simulink model "gm_HSG"  (R2017b)
settings: Solver=FixedStepDiscrete  StartTime=0.0  StopTime=Ts_240p  RelTol=1e-3
InitFcn:
  | Ts = 1e-3;
  | Ts_240p = 402*324*Ts;
undefined symbols (not defined in the file): gray, Rec, SDTV
libraries: hdlsllib x15, visionhdlfilter x8, simulink x3, visionhdlio x2, visionhdlconversions x1, visionhdlanalysis x1, dspvision x1
settings Model: ModifiedByFormat=4mbilal@gmail.com  Creator=The MathWorks, Inc.  LastModifiedBy=4mbilal@gmail.com
settings DataIOCC: LimitDataPoints=on  SaveFormat=Array  SaveOutput=off  SaveTime=off
settings OptimizationCC: BlockReduction=off  ConditionallyExecuteInputs=off  DefaultParameterBehavior=Inlined  LifeSpan=inf
settings DebuggingCC: AlgebraicLoopMsg=error  SolverPrmCheckMsg=warning  InheritedTsInSrcMsg=none  SingleTaskRateTransMsg=error  ParameterPrecisionLossMsg=none  AllowSymbolicDim=off  SFUnexpectedBacktrackingDiag=warning  SFNoUnconditionalDefaultTransitionDiag=warning  SFExecutionAtInitializationDiag=none  IntegerSaturationMsg=none
settings HardwareCC: ProdBitPerPointer=32  ProdBitPerSizeT=32  ProdBitPerPtrDiffT=32  ProdLargestAtomicFloat=None  ProdIntDivRoundTo=Undefined  ProdEndianess=Unspecified  ProdWordSize=32  ProdHWDeviceType=ASIC/FPGA->ASIC/FPGA  ProdEqTarget=off
settings ModelReferenceCC: PropagateSignalLabelsOutOfModel=off
settings CodeAppCC: StateflowObjectComments=on
settings GRTTargetCC: TargetLangStandard=C89/C90 (ANSI)  GeneratePreprocessorConditionals=Disable all
settings ConfigComp: CovMetricSettings=dw  CovHtmlReporting=on  CovSaveCumulativeToWorkspaceVar=on  CovSaveSingleToWorkspaceVar=on  CovShowResultsExplorer=off  CovExternalEMLEnable=off  CovSFcnEnable=off

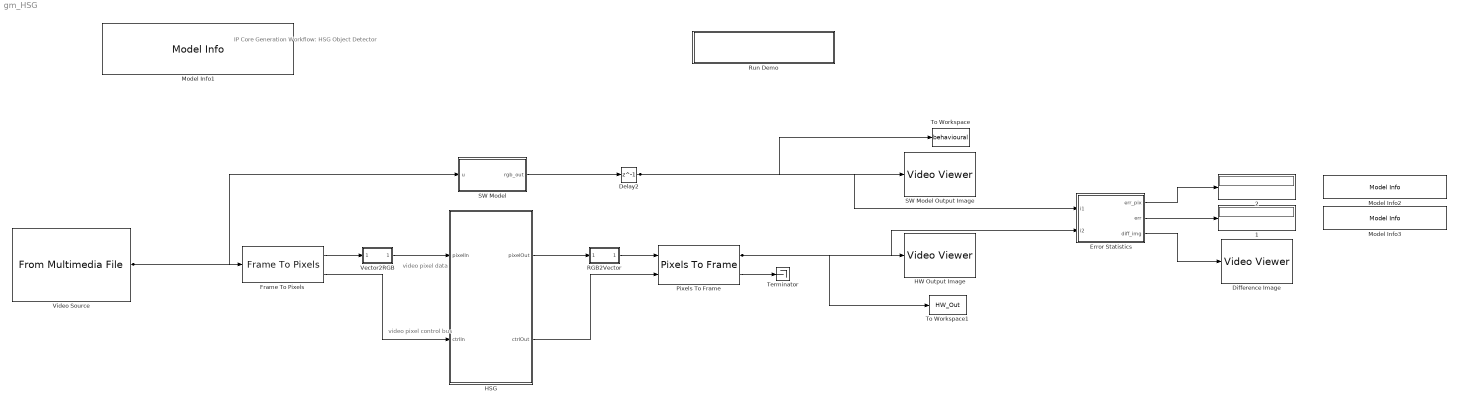
== system gm_HSG ==
  note: video pixel control bus
  note: IP Core Generation Workflow: HSG Object Detector
  note: video pixel data
  " 1" : Display
  " 2" : Display
  Delay2 : Delay  DelayLength=1  InitialCondition=0
  Difference Image : VideoViewer  colormapValue=gray(256)  FigPos=[516.2 717.2 730.4 340.8]
  Error Statistics : MATLAB Function  TreatAsAtomicUnit=on
  Frame To Pixels : visionhdlio/Frame To Pixels  NumComponents=3  VideoFormat=240p  ActivePixelsPerLine=32  ActiveVideoLines=18  TotalPixelsPerLine=42  TotalVideoLines=28  StartingActiveLine=6  FrontPorch=5  SampleTime=0
      settings: SourceProductName=Vision HDL Toolbox  SourceProductBaseCode=VT
  HSG : Subsystem  TreatAsAtomicUnit=on
  HW Output Image : VideoViewer  colormapValue=gray(256)  FigPos=[21.8 576.4 730.4 446.4]
  Model Info1 : simulink/Model-Wide Utilities/Model Info  Frame=on  DisplayStringWithTags=|  HorizontalTextAlignment=Center  LeftAlignmentValue=0.5
      | This Simulink model serves as the "High Level"
      |  framework for training, testing and HDL IP Core
      |  generation for video based object detection using
      |  HSG as the main feature.
  Model Info2 : simulink/Model-Wide Utilities/Model Info  Frame=on  DisplayStringWithTags=Percentage of Pixels with error  HorizontalTextAlignment=Center  LeftAlignmentValue=0.5
  Model Info3 : simulink/Model-Wide Utilities/Model Info  Frame=on  DisplayStringWithTags=Average error value per pixel  HorizontalTextAlignment=Center  LeftAlignmentValue=0.5
  Pixels To Frame : visionhdlio/Pixels To Frame  NumComponents=3  VideoFormat=240p  ActivePixelsPerLine=32  ActiveVideoLines=18  TotalPixelsPerLine=42  TotalVideoLines=28
      settings: SourceProductName=Vision HDL Toolbox  SourceProductBaseCode=VT
  RGB2Vector : Subsystem
  Run Demo : Subsystem
      settings: OpenFcn=hdladvisor([bdroot, '/HSG'])
      mask Display: disp('Launch HDL Workflow Advisor')
  SW Model : MATLAB Function  TreatAsAtomicUnit=on
  SW Model Output Image : VideoViewer  colormapValue=gray(256)  FigPos=[733.8 573.2 730.4 446.4]
  Terminator : Terminator
  To Workspace : ToWorkspace  VariableName=behavioural  SaveFormat=Timeseries  SampleTime=-1
  To Workspace1 : ToWorkspace  VariableName=HW_Out  SaveFormat=Timeseries  SampleTime=-1
  Vector2RGB : Subsystem
  Video Source : dspvision/From Multimedia File  inputFilename=E:\RnD\Current_Projects\Musawwir\Frameworks\HW\Musawwir_HW_Zedboard\Custom_IP_Cores\Matlab\HSG\engine_small.png  loop=on  numPlays=inf  outputStreams=Video only  videoDataType=uint8  audioDataType=int16  inheritSampleTime=off  userDefinedSampleTime=Ts_240p  noAudioOutput=off  isIntensityVideo=off  fourcc=RGB  colorVideoFormat=One multidimensional signal  outputEOF=off  dataOrg=Column-major  audioFrameSize=1024  computeAudioFrameSize=off  outSamplingMode=Sample based
      settings: SourceProductBaseCode=VP
  wires:
  Error Statistics/1(err_pix) -> " 2"/1
  Error Statistics/3(diff_img) -> Difference Image/1
  Delay2/1 -> SW Model Output Image/1, To Workspace/1, Error Statistics/1(i1)
  SW Model/1(rgb_out) -> Delay2/1
  Error Statistics/2(err) -> " 1"/1
  Pixels To Frame/1 -> HW Output Image/1, To Workspace1/1, Error Statistics/2(i2)
  Video Source/1 -> Frame To Pixels/1, SW Model/1(u)
  RGB2Vector/1(RGBVector) -> Pixels To Frame/1
  Frame To Pixels/2 -> HSG/2(ctrlIn)
  HSG/2(ctrlOut) -> Pixels To Frame/2
  Frame To Pixels/1 -> Vector2RGB/1(RGBVector)
  HSG/1(pixelOut) -> RGB2Vector/1(RGB)
  Vector2RGB/1(RGB) -> HSG/1(pixelIn)
  Pixels To Frame/2 -> Terminator/1

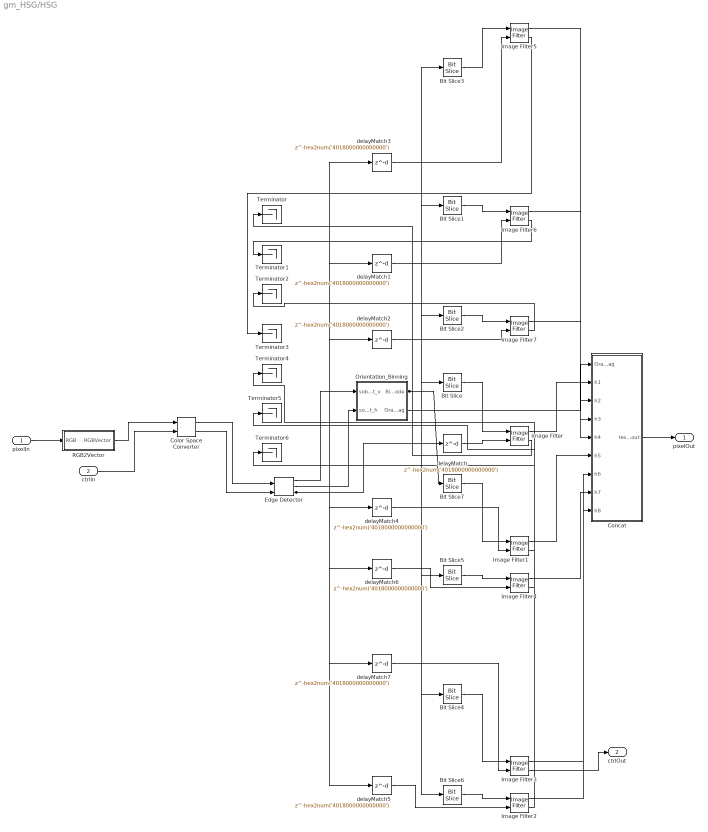
== system gm_HSG/HSG ==
  pixelIn : Inport  OutDataTypeStr=uint32  SampleTime=0.001
  ctrlIn : Inport  Port=2  SampleTime=0.001
  Bit Slice : hdlsllib/Logic and Bit Operations/Bit Slice  lidx=hex2num('401c000000000000')  ridx=hex2num('401c000000000000')
  Bit Slice1 : hdlsllib/Logic and Bit Operations/Bit Slice  lidx=hex2num('4018000000000000')  ridx=hex2num('4018000000000000')
  Bit Slice2 : hdlsllib/Logic and Bit Operations/Bit Slice  lidx=hex2num('4014000000000000')  ridx=hex2num('4014000000000000')
  Bit Slice3 : hdlsllib/Logic and Bit Operations/Bit Slice  lidx=hex2num('4010000000000000')  ridx=hex2num('4010000000000000')
  Bit Slice4 : hdlsllib/Logic and Bit Operations/Bit Slice  lidx=hex2num('0000000000000000')  ridx=hex2num('0000000000000000')
  Bit Slice5 : hdlsllib/Logic and Bit Operations/Bit Slice  lidx=hex2num('3ff0000000000000')  ridx=hex2num('3ff0000000000000')
  Bit Slice6 : hdlsllib/Logic and Bit Operations/Bit Slice  lidx=hex2num('4000000000000000')  ridx=hex2num('4000000000000000')
  Bit Slice7 : hdlsllib/Logic and Bit Operations/Bit Slice  lidx=hex2num('4008000000000000')  ridx=hex2num('4008000000000000')
  Color Space Converter : visionhdlconversions/Color Space Converter  Conversion=RGB to intensity  ConversionStandard=Rec. 601 (SDTV)  ScanningStandard=1250/50/2:1  SimulateUsing=Code generation
      settings: SourceProductName=Vision HDL Toolbox  SourceProductBaseCode=VT
  Concat : Subsystem
  Edge Detector : visionhdlanalysis/Edge Detector  Method=Sobel  BinaryImageOutputPort=off  GradientComponentOutputPorts=on  ThresholdSource=Input port  Threshold=20  LineBufferSize=1024  SimulateUsing=Code generation  roundingMode=Floor  overflowMode=off  GradientMin=[]  GradientMax=[]
      settings: SourceProductName=Vision HDL Toolbox  SourceProductBaseCode=VT
  Image Filter{,1..7} (8 alike) : visionhdlfilter/Image Filter  Coefficients="[ 1, 1, 1, 1, 1, 1;  1, 1, 1, 1, 1, 1; 1, 1, 1, 1, 1, 1; 1, 1, 1, 1, 1, 1; 1, 1, 1, 1, 1, 1; 1, 1, 1, 1, 1, 1]"  PaddingMethod=Constant  PaddingValue=0  LineBufferSize=1024  SimulateUsing=Code generation  roundingMode=Floor  overflowMode=on  CoeffMin=[]  CoeffMax=[]  OutputDataTypeStr=fixdt(0,4,0, 'DataTypeOverride', 'Off')  OutputMin=[]  OutputMax=[]
      settings: SourceProductName=Vision HDL Toolbox  SourceProductBaseCode=VT
  Orientation_Binning : Subsystem
  RGB2Vector : Subsystem
  Terminator{,1..6} (7 alike) : Terminator
  delayMatch{,1..7} (8 alike) : Delay  DelayLength=hex2num('4018000000000000')  InitialCondition=0  InputProcessing=Inherited  SampleTime=0.001
  pixelOut : Outport
  ctrlOut : Outport  Port=2
  wires:
  pixelIn/1 -> RGB2Vector/1(RGB)
  ctrlIn/1 -> Color Space Converter/2
  Bit Slice/1 -> Image Filter/1
  Bit Slice1/1 -> Image Filter6/1
  Bit Slice2/1 -> Image Filter7/1
  Bit Slice3/1 -> Image Filter5/1
  Bit Slice4/1 -> Image Filter3/1
  Bit Slice5/1 -> Image Filter4/1
  Bit Slice6/1 -> Image Filter2/1
  Bit Slice7/1 -> Image Filter1/1
  Color Space Converter/1 -> Edge Detector/1
  Color Space Converter/2 -> Edge Detector/2
  Concat/1(test_out) -> pixelOut/1
  Edge Detector/1 -> Orientation_Binning/1(sobel_gradient_v)
  Edge Detector/2 -> Orientation_Binning/2(sobel_gradient_h)
  delayMatch/1 -> Image Filter/2
  Image Filter/1 -> Concat/2(h1)
  Image Filter/2 -> Terminator/1
  Image Filter1/1 -> Concat/6(h5)
  Image Filter1/2 -> Terminator4/1
  Image Filter2/1 -> Concat/7(h6)
  Image Filter2/2 -> Terminator5/1
  Image Filter3/1 -> Concat/9(h8)
  Image Filter3/2 -> ctrlOut/1
  Image Filter4/1 -> Concat/8(h7)
  Image Filter4/2 -> Terminator6/1
  Image Filter5/1 -> Concat/5(h4)
  Image Filter5/2 -> Terminator3/1
  Image Filter6/1 -> Concat/3(h2)
  Image Filter6/2 -> Terminator1/1
  Image Filter7/1 -> Concat/4(h3)
  Image Filter7/2 -> Terminator2/1
  Orientation_Binning/1(Bin_Code) -> Bit Slice7/1, Bit Slice6/1, Bit Slice5/1, Bit Slice4/1, Bit Slice3/1, Bit Slice2/1, Bit Slice1/1, Bit Slice/1
  Orientation_Binning/2(Grad_Mag) -> Concat/1(Grad_Mag)
  RGB2Vector/1(RGBVector) -> Color Space Converter/1
  delayMatch1/1 -> Image Filter6/2
  delayMatch2/1 -> Image Filter7/2
  delayMatch3/1 -> Image Filter5/2
  delayMatch4/1 -> Image Filter1/2
  delayMatch5/1 -> Image Filter2/2
  delayMatch6/1 -> Image Filter4/2
  delayMatch7/1 -> Image Filter3/2
  Edge Detector/3 -> delayMatch7/1, delayMatch6/1, delayMatch5/1, delayMatch4/1, delayMatch3/1, delayMatch2/1, delayMatch1/1, delayMatch/1

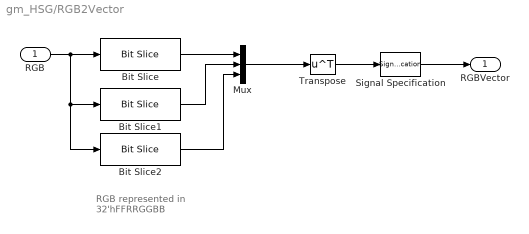
== system gm_HSG/RGB2Vector ==
  note: RGB represented in
      | 32'hFFRRGGBB
  RGB : Inport
  Bit Slice : hdlsllib/Logic and Bit Operations/Bit Slice  lidx=23  ridx=16
  Bit Slice1 : hdlsllib/Logic and Bit Operations/Bit Slice  lidx=15  ridx=8
  Bit Slice2 : hdlsllib/Logic and Bit Operations/Bit Slice  lidx=7  ridx=0
  Mux : Mux  Inputs=3
  Signal Specification : SignalSpecification
  Transpose : Math  Operator=transpose  SaturateOnIntegerOverflow=on
  RGBVector : Outport
  wires:
  Signal Specification/1 -> RGBVector/1
  Transpose/1 -> Signal Specification/1
  RGB/1 -> Bit Slice/1, Bit Slice1/1, Bit Slice2/1
  Bit Slice1/1 -> Mux/2
  Bit Slice2/1 -> Mux/3
  Bit Slice/1 -> Mux/1
  Mux/1 -> Transpose/1

== system gm_HSG/Run Demo ==

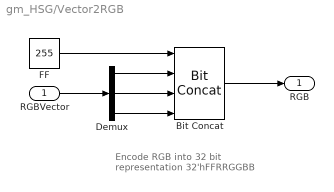
== system gm_HSG/Vector2RGB ==
  note: Encode RGB into 32 bit representation
      | 32'hFFRRGGBB
  RGBVector : Inport
  Bit Concat : hdlsllib/Logic and Bit Operations/Bit Concat  numInputs=4
      settings: SourceProductName=HDL Coder  SourceProductBaseCode=HD
  Demux : Demux  Outputs=3
  FF : Constant  Value=255  OutDataTypeStr=uint8  SampleTime=Ts
  RGB : Outport
  wires:
  Demux/3 -> Bit Concat/4
  Demux/2 -> Bit Concat/3
  Demux/1 -> Bit Concat/2
  FF/1 -> Bit Concat/1
  RGBVector/1 -> Demux/1
  Bit Concat/1 -> RGB/1

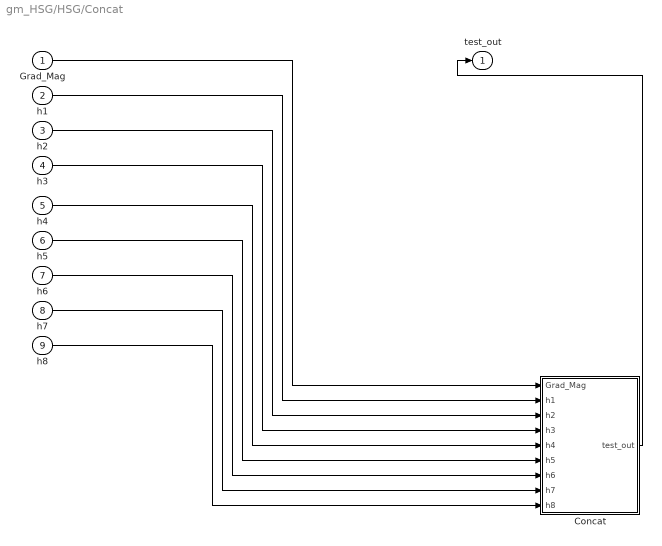
== system gm_HSG/HSG/Concat ==
  Grad_Mag : Inport  SampleTime=0.001
  h1 : Inport  Port=2  SampleTime=0.001
  h2 : Inport  Port=3  SampleTime=0.001
  h3 : Inport  Port=4  SampleTime=0.001
  h4 : Inport  Port=5  SampleTime=0.001
  h5 : Inport  Port=6  SampleTime=0.001
  h6 : Inport  Port=7  SampleTime=0.001
  h7 : Inport  Port=8  SampleTime=0.001
  h8 : Inport  Port=9  SampleTime=0.001
  Concat : MATLAB Function  TreatAsAtomicUnit=on
  test_out : Outport
  wires:
  Concat/1(test_out) -> test_out/1
  Grad_Mag/1 -> Concat/1(Grad_Mag)
  h1/1 -> Concat/2(h1)
  h2/1 -> Concat/3(h2)
  h3/1 -> Concat/4(h3)
  h4/1 -> Concat/5(h4)
  h5/1 -> Concat/6(h5)
  h6/1 -> Concat/7(h6)
  h7/1 -> Concat/8(h7)
  h8/1 -> Concat/9(h8)

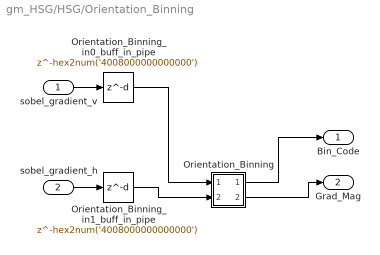
== system gm_HSG/HSG/Orientation_Binning ==
  sobel_gradient_v : Inport  SampleTime=0.001
  sobel_gradient_h : Inport  Port=2  SampleTime=0.001
  Orientation_Binning : Subsystem
  Orientation_Binning_in0_buff_in_pipe : Delay  DelayLength=hex2num('4008000000000000')  InitialCondition=0  InputProcessing=Inherited  SampleTime=0.001
  Orientation_Binning_in1_buff_in_pipe : Delay  DelayLength=hex2num('4008000000000000')  InitialCondition=0  InputProcessing=Inherited  SampleTime=0.001
  Bin_Code : Outport
  Grad_Mag : Outport  Port=2
  wires:
  Orientation_Binning/1(Out1) -> Bin_Code/1
  Orientation_Binning/2(Out2) -> Grad_Mag/1
  Orientation_Binning_in0_buff_in_pipe/1 -> Orientation_Binning/1(In1)
  Orientation_Binning_in1_buff_in_pipe/1 -> Orientation_Binning/2(In2)
  sobel_gradient_v/1 -> Orientation_Binning_in0_buff_in_pipe/1
  sobel_gradient_h/1 -> Orientation_Binning_in1_buff_in_pipe/1

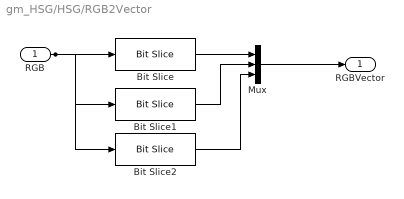
== system gm_HSG/HSG/RGB2Vector ==
  RGB : Inport  SampleTime=0.001
  Bit Slice : hdlsllib/Logic and Bit Operations/Bit Slice  lidx=23  ridx=16
  Bit Slice1 : hdlsllib/Logic and Bit Operations/Bit Slice  lidx=15  ridx=8
  Bit Slice2 : hdlsllib/Logic and Bit Operations/Bit Slice  lidx=7  ridx=0
  Mux : Mux  Inputs=3
  RGBVector : Outport
  wires:
  Bit Slice/1 -> Mux/1
  Bit Slice1/1 -> Mux/2
  Bit Slice2/1 -> Mux/3
  Mux/1 -> RGBVector/1
  RGB/1 -> Bit Slice2/1, Bit Slice1/1, Bit Slice/1

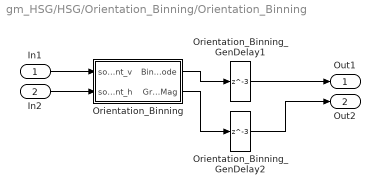
== system gm_HSG/HSG/Orientation_Binning/Orientation_Binning ==
  In1 : Inport
  In2 : Inport  Port=2
  Orientation_Binning : MATLAB Function  TreatAsAtomicUnit=on
  Orientation_Binning_GenDelay1 : Delay  DelayLength=3  InputProcessing=Inherited
  Orientation_Binning_GenDelay2 : Delay  DelayLength=3  InputProcessing=Inherited
  Out1 : Outport
  Out2 : Outport  Port=2
  wires:
  In1/1 -> Orientation_Binning/1(sobel_gradient_v)
  In2/1 -> Orientation_Binning/2(sobel_gradient_h)
  Orientation_Binning/1(Bin_Code) -> Orientation_Binning_GenDelay1/1
  Orientation_Binning_GenDelay1/1 -> Out1/1
  Orientation_Binning/2(Grad_Mag) -> Orientation_Binning_GenDelay2/1
  Orientation_Binning_GenDelay2/1 -> Out2/1

== matlab function gm_HSG/SW Model ==
  data: u input; rgb_out output
function rgb_out   = HSG_SW(u)
%   Convert to Graysclae
y = double(rgb2gray(u));
s = size(y);

%   Apply Soble filter in both vertical and horizontal directions
v = 0.125*[1,0,-1;2,0,-2;1,0,-1];
h = 0.125*[1,2,1;0,0,0;-1,-2,-1];
Sobel_v = imfilter(y,v);
Sobel_h = imfilter(y,h);

%   Calculate Gradient magnitude and orientation
Grad_Mag = uint8(sqrt(double(Sobel_v.*Sobel_v + Sobel_h.*Sobel_h)));
Grad_Or = atan2(Sobel_v,Sobel_h);
for i=1:240,        %Keep only unsigned edges [0 180]
    for j=1:320,
        if(Grad_Or(i,j)<0)
            Grad_Or(i,j) = Grad_Or(i,j) + pi;
        end
    end
end

%   Calculate Orientation bin number
n = 8;  %No. of bins
% Bin_index = zeros(240,320,1);
Bin_index = 2.^floor(Grad_Or*n/pi);      %One-hot encoding for histogram population using adder-filters

%   Fill orientation histograms
Significance = (Grad_Mag>16);
G0 = double((Bin_index==1)   &   Significance);
G1 = double((Bin_index==2)   &   Significance);
G2 = double((Bin_index==4)   &   Significance);
G3 = double((Bin_index==8)   &   Significance);
G4 = double((Bin_index==16)  &   Significance);
G5 = double((Bin_index==32)  &   Significance);
G6 = double((Bin_index==64)  &   Significance);
G7 = double((Bin_index==128) &   Significance);
%   Build histograms using sum filter
f = ones(6,6);
OH0 = imfilter(G0,f);
OH1 = imfilter(G1,f);
OH2 = imfilter(G2,f);
OH3 = imfilter(G3,f);
OH4 = imfilter(G4,f);
OH5 = imfilter(G5,f);
OH6 = imfilter(G6,f);
OH7 = imfilter(G7,f);
%   Saturate to 15
OH0(OH0>15) = 15;
OH1(OH1>15) = 15;
OH2(OH2>15) = 15;
OH3(OH3>15) = 15;
OH4(OH4>15) = 15;
OH5(OH5>15) = 15;
OH6(OH6>15) = 15;
OH7(OH7>15) = 15;

%   Prepare the signal for display using RGB componnets
rgb = zeros(240,320,3);

%Uncomment for Grayscale Image Output
% rgb(:,:,1) = y;
% rgb(:,:,2) = y;
% rgb(:,:,3) = y;

%Uncomment for Gradient Image Output
% rgb(:,:,1) = Grad_Mag;
% rgb(:,:,2) = Grad_Mag;
% rgb(:,:,3) = Grad_Mag;

%Uncomment for Gradient Image Output
% rgb(:,:,1) = Bin_index;
% rgb(:,:,2) = Bin_index;
% rgb(:,:,3) = Bin_index;

%Uncomment for Histogram Image Output
FRGB_Vector = OH7 + OH6*(2^4) + OH5*(2^8) + OH4*(2^12) + OH3*(2^16) + OH2*(2^20) + OH1*(2^24) + OH0*(2^28);
F = floor(FRGB_Vector/2^24);
RGB_Vector = FRGB_Vector - F*2^24;
R = floor(RGB_Vector/2^16);
GB_Vector = RGB_Vector - R*2^16;
G = floor(GB_Vector/2^8);
B = GB_Vector - G*2^8;

rgb(:,:,1) = R;
rgb(:,:,2) = G;
rgb(:,:,3) = B;

%   RGB signal output
rgb_out = uint8(rgb);

== matlab function gm_HSG/HSG/Concat/Concat ==
  data: Grad_Mag input; h1 input; test_out output; h2 input; h3 input; h4 input; h5 input; h6 input; h7 input; h8 input
function test_out  = Concat(Grad_Mag, h1, h2, h3, h4, h5, h6, h7, h8)

h1_in = double(h1);
h2_in = double(h2);
h3_in = double(h3);
h4_in = double(h4);
h5_in = double(h5);
h6_in = double(h6);
h7_in = double(h7);
h8_in = double(h8);

h11 = fi(h1_in, 0, 4, 0);
h22 = fi(h2_in, 0, 4, 0);
h33 = fi(h3_in, 0, 4, 0);
h44 = fi(h4_in, 0, 4, 0);
h55 = fi(h5_in, 0, 4, 0);
h66 = fi(h6_in, 0, 4, 0);
h77 = fi(h7_in, 0, 4, 0);
h88 = fi(h8_in, 0, 4, 0);

test_out = bitconcat(h88,h77,h66,h55,h44,h33,h22,h11);

== matlab function gm_HSG/HSG/Orientation_Binning/Orientation_Binning/Orientation_Binning ==
  data: sobel_gradient_v input; sobel_gradient_h input; Bin_Code output; Grad_Mag output
function [Bin_Code, Grad_Mag] = Orientation_Binning(sobel_gradient_v, sobel_gradient_h)
    Alpha = fi(255, 0, 8, 0);

    %No real need for square root operation. Use condition Grad_Mag > 256
    %instead of Grad_Mag > 16.
%     Grad_Mag = sqrt(sobel_gradient_v*sobel_gradient_v + sobel_gradient_h*sobel_gradient_h);
    Grad_Mag = (sobel_gradient_v*sobel_gradient_v + sobel_gradient_h*sobel_gradient_h);
       
    dy = sobel_gradient_v;
    dx = sobel_gradient_h;
    if(dy<0)        %Use only [0 180] range (unsigned orientation)
        dy = -dy;
        dx = -dx;
    else
        dy = dy;
        dx = dx;
    end
    
    B = [0.41421356  1   2.41421356];     %Bin boundaries for 8 bin scheme
    
%     %Approximate binning: No interpolation
    dxp = -dx;
    if(Grad_Mag > 256)
        if(dx >= 0)
            if(dy < dx*B(1))
                Bin_index = 1;
            elseif(dy < dx*B(2))
                Bin_index = 2;
            elseif(dy < dx*B(3))
                Bin_index = 4;
            else
                Bin_index = 8;
            end
        else
            if(dy < dxp*B(1))
                Bin_index = 128;
            elseif(dy < dxp*B(2))
                Bin_index = 64;
            elseif(dy < dxp*B(3))
                Bin_index = 32;
            else
                Bin_index = 16;
            end
        end
    else
        Bin_index = 0;
    end

    Bin_Code = fi(Bin_index, 0, 8, 0);

%     red = 100;
%     green = 100;
%     blue = 100;
%     if(Grad_Mag<16)
%         red = 0;
%         green = 0;
%         blue = 0;
%     else
%         if(Bin_index == 1)
%             red = red + 100;
%         elseif(Bin_index == 2)
%         green = green + 100;
%     elseif(Bin_index == 3)
%         red = red + 100;
%         green = green + 100;
%     elseif(Bin_index == 4)
%         blue = blue + 100;
%     elseif(Bin_index == 5)
%         red = red + 100;
%         blue = blue + 100;
%     elseif(Bin_index == 6)
%         green = green + 100;
%         blue = blue + 100;
%     elseif(Bin_index == 7)
%         red = red + 100;
%         green = green + 50;
%     elseif(Bin_index == 8)
%         green = green + 50;
%         blue = blue + 75;
%     end
        
%     r = fi(red, 0, 8, 0);
%     g = fi(green, 0, 8, 0);
%     b = fi(blue, 0, 8, 0);
    
%     r = fi(Bin_index, 0, 8, 0);
%     g = fi(Bin_index, 0, 8, 0);
%     b = fi(Bin_index, 0, 8, 0);
%     
%     
%     Sig_Out = bitconcat(Alpha,r,g,b);

== matlab function gm_HSG/Error Statistics ==
  data: err_pix output; i1 input; err output; i2 input; diff_img output
function [err_pix, err, diff_img] = Error_Stats(i1,i2)
e = i1-i2;
diff_img = abs(e);
e = e(:);
z = (e==0);     %Pixels with zero error
err_pix = 100*(1-sum(z)/length(z)); %Percentage of pixels with error
err = sum(sum(sum(abs(e))));    %Sum of all error values
err = err/length(z);            %Average error per pixel
